simulink model "SimpleBot_V3"  (R2024a)
settings: Solver=ode45  StartTime=0.0  StopTime=10.0  RelTol=1e-3
values from neighbouring files (symbols this model uses):
  Achsabstand = 0.15    [Model1Sensibilities.m]    (also in Model1numericalPSA.m; Model2Sensibilities.m; Modellvalidierung.m; MotorSens2.m)
  B_dis = 0.25    [Model1Sensibilities.m]    (also in Model1numericalPSA.m = 0.15; Model2Sensibilities.m; Modellvalidierung.m = 0.15; MotorSens2.m)
  g = 9.81    [Model1Sensibilities.m]    (also in Model1numericalPSA.m; Model2Sensibilities.m; Modellvalidierung.m; MotorSens2.m)
  I_Bot = 0.0072    [Model1Sensibilities.m]    (also in Model1numericalPSA.m; Model2Sensibilities.m; Modellvalidierung.m; MotorSens2.m)
  m_ges = 1    [Model1Sensibilities.m]    (also in Model1numericalPSA.m; Model2Sensibilities.m; Modellvalidierung.m; MotorSens2.m)
  Reifen_Radius = 0.04    [Model1Sensibilities.m]    (also in Model1numericalPSA.m; Model2Sensibilities.m; Modellvalidierung.m; MotorSens2.m)
  Xi = 2/3    (= 0.666666666667)    [Model1Sensibilities.m]    (also in Model1numericalPSA.m = 0.333333333333; Model2Sensibilities.m; Modellvalidierung.m = 0.333333333333; MotorSens2.m)
settings Model: Creator=jakob  LastModifiedBy=Jakob Reindl

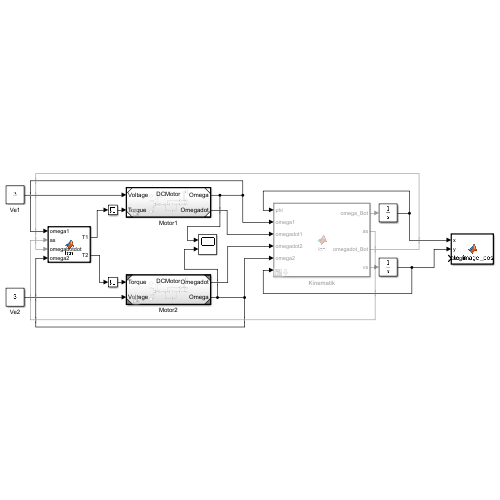
[thumbnail: Simulink's stored preview of the top-level diagram]
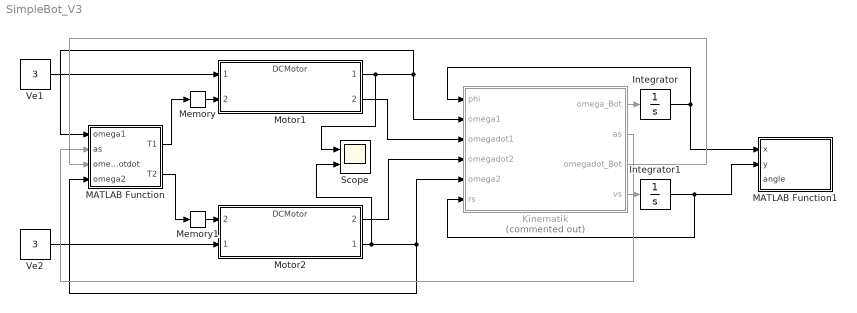
== system SimpleBot_V3 ==
  Integrator : Integrator
  Integrator1 : Integrator
  Kinematik : MATLAB Function  Commented=on  TreatAsAtomicUnit=on  mask{B_dis=B_dis, Achsabstand=Achsabstand, Reifen_Radius=Reifen_Radius, Xi=Xi}
      mask prompts: B_dis "Distance from rear block to axis"; Reifen_Radius "Reifenradius"
  MATLAB Function : MATLAB Function  TreatAsAtomicUnit=on
  MATLAB Function1 : MATLAB Function  TreatAsAtomicUnit=on
  Memory : Memory  InitialCondition=3.466
  Memory1 : Memory  InitialCondition=3.466
  Motor1 : ModelReference  ModelNameDialog=DCMotor  SimulationMode=Normal  ModelReferenceVersion=1.6
  Motor2 : ModelReference  ModelNameDialog=DCMotor  SimulationMode=Normal  ModelReferenceVersion=1.6
      settings: PortSchema="{\"entries\":[{\"content\":{\"sides\":[{\"content\":{\"connectorIds\":[\"In2\",\"In1\"]},\"type\":\"ConnectorPlacement.EquallySpacedRectSide\",\"uuid\":\"a74839e0-9594-4d91-a47a-bf9c9b4b98c9\"},{\"content\":{\"connectorIds\":[\"Out2\",\"Out1\"],\"side\":\"RIGHT\"},\"type\":\"ConnectorPlacement.EquallySpacedRectSide\",\"uuid\":\"51af5672-9c33-4899-a42f-4b737d1c3e1f\"},{\"content\":{\"side\":\"TOP\"},\"type\":\"ConnectorPlacement.EquallySpacedRectSide\",\"uuid\":\"938b8719-7670-4eda-aa86-bdd9d1e4edbf\"}]},\"type\":\"ConnectorPlacement.EquallySpacedConnector\",\"uuid\":\"899e2604-6c92-4fa5-991d-253a33e61c0b\"}],\"packageUris\":[\"http://schema.mathworks.com/mf0/Connector/R2020b\"],\"version\":\"1.0\"}"
  Scope : Scope  NumInputPorts=2
  Ve1 : Constant  Value=3
  Ve2 : Constant  Value=3
  wires:
  Ve1/1 -> Motor1/1
  Ve2/1 -> Motor2/1
  Motor1/1 -> Kinematik/2(omega1), MATLAB Function/1(omega1), Scope/1
  Motor2/1 -> Scope/2, Kinematik/5(omega2), MATLAB Function/4(omega2)
  Kinematik/1(omega_Bot) -> Integrator/1
  Integrator/1 -> MATLAB Function1/1(x), Kinematik/1(phi)
  Motor1/2 -> Kinematik/3(omegadot1)
  Motor2/2 -> Kinematik/4(omegadot2)
  Kinematik/4(vs) -> Integrator1/1
  Integrator1/1 -> Kinematik/6(rs), MATLAB Function1/2(y)
  Kinematik/2(as) -> MATLAB Function/2(as)
  Kinematik/3(omegadot_Bot) -> MATLAB Function/3(omegabotdot)
  MATLAB Function/1(T1) -> Memory/1
  MATLAB Function/2(T2) -> Memory1/1
  Memory/1 -> Motor1/2
  Memory1/1 -> Motor2/2

== matlab function SimpleBot_V3/MATLAB Function ==
  data: omega1 input; as input; omegabotdot input; omega2 input; T1 output; T2 output; I_Bot parameter; g parameter; m_ges parameter; B_dis parameter; Reifen_Radius parameter; Achsabstand parameter; Xi parameter
function [T1, T2] = fcn(omega1,as,omegabotdot, omega2,I_Bot, g, m_ges, B_dis, Reifen_Radius, Achsabstand, Xi)
%Formeln in Notizen übersichtlicher!

%Berechnung-Kraftrichtung-Block-Reibkräfte-> Alpha
%Geschwindigkeitspol xp
xp = (Achsabstand/2) * ((omega1 *Reifen_Radius + omega2 * Reifen_Radius)/(omega2 * Reifen_Radius-omega1 *Reifen_Radius));
%Berechnung-Winkel
alpha = atan(B_dis / xp);

%Brechnung-Boden-Kontakt-Kräfte

Fg_Bot = m_ges * g;                 %Schwerpunkt bekannt
%F_Reifen = Fg_Bot * ((1-Xi)/2);
F_Block = Fg_Bot * (Xi/2);

%Brechung der Lastmomente T1 & T2

T1 = -(Reifen_Radius/2)* (m_ges * as - (2/Achsabstand)* I_Bot * omegabotdot - F_Block * (2*cos(alpha) + (4/Achsabstand)*B_dis*sin(alpha)*(1-Xi)));

T2 = -(Reifen_Radius/2)* (m_ges * as + (2/Achsabstand)* I_Bot * omegabotdot - F_Block * (2*cos(alpha) - (4/Achsabstand)*B_dis*sin(alpha)*(1-Xi)));

== matlab function SimpleBot_V3/Kinematik ==
  data: phi input; omega1 input; omegadot1 input; omegadot2 input; omega2 input; rs input; omega_Bot output; as output; omegadot_Bot output; vs output; B_dis parameter; Achsabstand parameter; Reifen_Radius parameter; Xi parameter
function [omega_Bot, as, omegadot_Bot, vs]= fcn(phi, omega1, omegadot1,omegadot2, omega2,  rs, B_dis, Achsabstand, Reifen_Radius, Xi)

%omega1 = 2 ;
%omega2 = 7;
%omegadot1 = 3;
%omegadot2 = 1;
%phi = 30;
%rs = [0;0];
omega_GB1 = Motoruebersetzung * omega1;
omega_GB2 = Motoruebersetzung * omega2;

RotPhi = [cosd(phi) -sind(phi); sind(phi) cosd(phi)];

r10 = rs + RotPhi * [-B_dis*Xi; Achsabstand/2];
r20 = rs + RotPhi * [-B_dis*Xi ; -Achsabstand/2];

v10 = RotPhi * [1;0] * omega_GB1 * Reifen_Radius;
v20 = RotPhi * [1;0] * omega_GB2 * Reifen_Radius;
vs = RotPhi * [1;0] * ((omega_GB1 * Reifen_Radius + omega_GB2 * Reifen_Radius)/2);

o_numerator = (v20(1) - v10(1)) * (r10(2) - r20(2)) + (v20(2) - v10(2)) * (r20(1) - r10(1));
o_denominator = (r10(2) - r20(2))^2 + (r20(1) - r10(1))^2;
omega_Bot = o_numerator / o_denominator;

a10 = RotPhi * [1;0] * omegadot1 * Reifen_Radius;
a20 = RotPhi * [1;0] * omegadot2 * Reifen_Radius;
as = RotPhi * [1;0] * ((omegadot1 * Reifen_Radius + omegadot2 * Reifen_Radius)/2);

odot_numerator = (a20(1) - a10(1) - omega_Bot^2 * (r10(1) - r20(1))) * (r10(2) - r20(2)) + (a20(2) - a10(2) - omega_Bot^2 * (r10(2) - r20(2))) * (r20(1) - r10(1));
odot_denominator = (r10(2) - r20(2))^2 + (r20(1) - r10(1))^2;
omegadot_Bot = odot_numerator/odot_denominator;

== matlab function SimpleBot_V3/MATLAB Function1 ==
  data: x input; y input; angle input
function update_image_position(x,y, angle)
    % MATLAB GUI erstellen
    f = uifigure('Name', 'Bildposition');
    ax = axes(f);
    img = imread('Bot-Bild.jpg');
    
    % Rotation und Positionierung des Bildes
    img_rot = imrotate(img, angle); % Bild rotieren
    
    % Das Bild in der GUI anzeigen
    imshow(img_rot, 'Parent', ax);
    % Position des Bildes anpassen
    set(ax, 'XLim', [x, x + size(img_rot,2)]);
    set(ax, 'YLim', [y, y + size(img_rot,1)]);
end
